simulink model "new_foc_mmd"  (R2024b)
settings: Solver=VariableStepAuto  StartTime=0.0  StopTime=3.14  FixedStep=0.000001  MaxStep=1e-4  RelTol=1e-3
model workspace (MAT data in the model file):
  fs = 4000
undefined symbols (not defined in the file): speed_ref, Ts
libraries: simulink x13, spsIGBTDiodeLib x6, slpidlib x3, spsVoltageMeasurementLib x3, spsPermanentMagnetSynchronousMachineLib x1, spsDCVoltageSourceLib x1, spsSawtoothGeneratorLib x1, simulink_extras x1, spsThreePhaseVIMeasurementLib x1, spspowerguiLib x1
(part 1 of 2)
settings Model: Creator=Admin  LastModifiedBy=INNAGOL2
settings SolverCC: ZeroCrossAlgorithm=Adaptive
settings DebuggingCC: MaskedZcDiagnostic=none  IgnoredZcDiagnostic=none
settings RTWCC: GPUComputeCapability=3.5

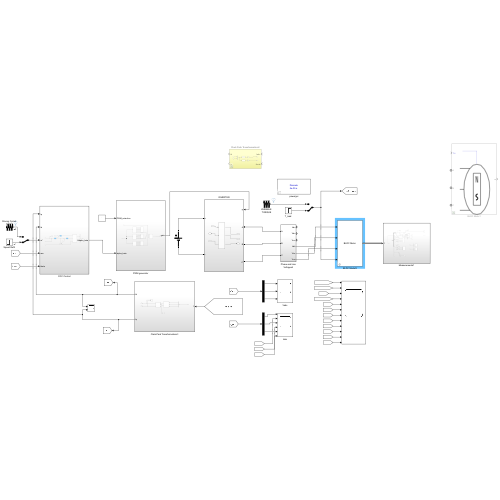
[thumbnail: Simulink's stored preview of the top-level diagram]
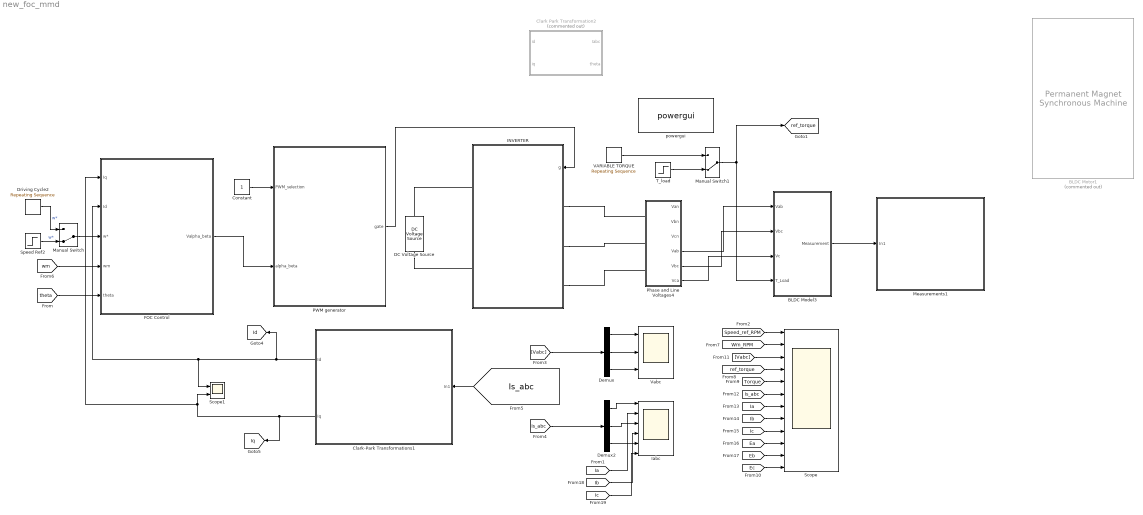
== system new_foc_mmd ==
  BLDC Model3 : Subsystem  mask(BLDC Motor :){Rs=0.7, Lls=2.7e-3, Phi_m=0.1194, J=0.0027, B=0.0004924, P=8}
      mask prompts: Rs "Resistance - Rs [ohms]"; Lls "Inductance - Lls [H]"; Phi_m "Rotor Flux [wb]"; J "Rotor Inertia - J [kg-m^2]"; B "Friction Coefficient -B"; P "No of Poles"
      mask init:
      | Trap=0.5;
      mask Display: fprintf('BLDC Motor')
  BLDC Motor1 : spsPermanentMagnetSynchronousMachineLib/Permanent Magnet Synchronous Machine  Commented=on  NbPhases=3  FluxDistribution=Trapezoidal  RotorType=Round  MechanicalLoad=Torque Tm  PresetModel=No  ShowDetailedParameters=on  MeasurementBus=off  Resistance=0.7  Inductance=2.7e-3  dqInductances=[8.5e-3,8.5e-3]  La=0.000835  MachineConstant=Flux linkage established by magnets (V.s)  Flux=0.1194  VoltageCst=100.0283  TorqueCst=0.9552  Flat=120  Mechanical=[0.0027 0.0004924 4]  PolePairs=4  InitialConditions=[0,0, 0,0]  InitialConditions5ph=[0 0 0 0 0 0]  RefAngle=Aligned with phase A axis (original Park)  IterativeDiscreteModel=Trapezoidal non iterative  TsBlock=-1  TsPowergui=0
  Clark Park Transformation2 : Subsystem  Commented=on
  Clark-Park Transformations1 : Subsystem
      settings: PortSchema="{\"entries\":[{\"content\":{\"sides\":[{\"content\":{\"connectorIds\":[\"Out1\",\"Out2\"]},\"type\":\"ConnectorPlacement.EquallySpacedRectSide\",\"uuid\":\"c290a13d-b4ce-440f-9d53-4b9274feb83f\"},{\"content\":{\"connectorIds\":[\"In1\"],\"side\":\"RIGHT\"},\"type\":\"ConnectorPlacement.EquallySpacedRectSide\",\"uuid\":\"3b8acf4d-0134-48df-ade6-fa9dd8548719\"},{\"content\":{\"side\":\"TOP\"},\"type\":\"ConnectorPlacement.EquallySpacedRectSide\",\"uuid\":\"08682ee2-bcb7-4f48-a64a-1997ed6d0a04\"}]},\"type\":\"ConnectorPlacement.EquallySpacedConnector\",\"uuid\":\"e640fd84-78ba-4bab-8695-1c4b1b64123a\"}],\"packageUris\":[\"http://schema.mathworks.com/mf0/Connector/R2020b\"],\"version\":\"1.0\"}"
  Constant : Constant
  DC Voltage Source : spsDCVoltageSourceLib/DC Voltage Source  Amplitude=160  Measurements=None
  Demux : Demux  Outputs=3
  Demux2 : Demux  Outputs=3
  Driving Cycle2 : simulink/Sources/Repeating Sequence  rep_seq_t=[0 1 2 3 4 5 6 7 8 9 10 11 11.0001 12 13]  rep_seq_y=[0 20 20 0 0 0 -30 -30 0 0 50 50 40 40 0]
  FOC Control : Subsystem
  INVERTER : Subsystem
  Iabc : Scope  NumInputPorts=6
  Manual Switch : ManualSwitch  CurrentSetting=0
  Manual Switch1 : ManualSwitch  CurrentSetting=0
  Measurements1 : Subsystem
  PWM generator : Subsystem
  Phase and Line Voltages4 : Subsystem
  Scope : Scope  NumInputPorts=12
  Scope1 : Scope  NumInputPorts=2
  Speed Ref2 : Step  Time=0.1  After=150  SampleTime=0
  "T_load " : Step  Time=0.1  After=5  SampleTime=0
  VARIABLE TORQUE : simulink/Sources/Repeating Sequence  rep_seq_t=[0 1 2 3 4 5 6 7 8 9 10 11 12 13]  rep_seq_y=[3 3 3 3 5 5 5 -2 -2 -2 1 1 1 1 ]
  Vabc : Scope  NumInputPorts=3
  powergui : spspowerguiLib/powergui  Priority=1  SimulationMode=Discrete  SampleTime=5e-05  frequency=60  Iterations=50  frequencyindice=0  Pbase=100e6  ErrMax=1e-4  UnitsV=kV  UnitsW=MW  buscounter=0  FunctionMessages=off  echomessages=off  EnableUseOfTLC=off  CurrentSourceSwitches=off  DisableSnubberDevices=off  DisableRonSwitches=off  DisableVfSwitches=off  DisplayEquations=off  AutomaticDiscreteSolvers=off  SolverType=Tustin/Backward Euler (TBE)  Interpol=off  ExternalGateDelay=off  methode=off  Ts=100  x0status=blocks  SPID=on  SwTol=0  HookPort=off  NonlinearTolerance=1e-4  nMaxIteration=100  ContinueOnMaxIteration=off  RestoreLinks=warning  ResistiveCurrentMeasurement=off  Frange=[0:2:500]  Ylog=off  Xlog=on  ShowGrid=off  save=off  variable=ZData  structure=0  ZoomFFT=off  StartTime=0.0  cycles=1  DisplayStyle=1  fundamental=60  FreqAxis=off  MaxFrequency=1000  frequencyindicesteady=1  RmsSteady=1  display=off
  tag scope: Id=global, Iq=global, ref_torque=global
  wires:
  Demux/3 -> Vabc/3
  Demux/1 -> Vabc/1
  Demux/2 -> Vabc/2
  Demux2/1 -> Iabc/1
  Demux2/2 -> Iabc/3
  Demux2/3 -> Iabc/5
  [Vabc] -> Demux/1
  [Is_abc] -> Demux2/1
  PWM generator/1(gate) -> INVERTER/1(g)
  [Is_abc] -> Clark-Park Transformations1/1(In1)
  Clark-Park Transformations1/1(Id) -> [Id], Scope1/1, FOC Control/2(Id)
  Clark-Park Transformations1/2(Iq) -> Scope1/2, FOC Control/1(Iq), [Iq]
  [wm] -> FOC Control/4(wm)
  [theta] -> FOC Control/5(theta)
  Constant/1 -> PWM generator/1(PWM_selection)
  FOC Control/1(Valpha_beta) -> PWM generator/2(alpha_beta)
  Speed Ref2/1 -> Manual Switch/2  "w*"
  Manual Switch/1 -> FOC Control/3(w*)
  VARIABLE TORQUE/1 -> Manual Switch1/1
  "T_load "/1 -> Manual Switch1/2
  Manual Switch1/1 -> BLDC Model3/4(T_Load), [ref_torque]
  Driving Cycle2/1 -> Manual Switch/1  "w*"
  [Vabc] -> Scope/3
  [Ib] -> Scope/8
  [Ia] -> Scope/7
  [Ea] -> Scope/10
  [ref_torque] -> Scope/4
  [Ic] -> Scope/9
  [Ec] -> Scope/12
  [Eb] -> Scope/11
  [Torque] -> Scope/5
  [Wm_RPM] -> Scope/2
  [Is_abc] -> Scope/6
  [Speed_ref_RPM] -> Scope/1
  [Ia] -> Iabc/2
  [Ib] -> Iabc/4
  [Ic] -> Iabc/6
  BLDC Model3/1(Measurement) -> Measurements1/1(In1)
  Phase and Line Voltages4/4(Vab) -> BLDC Model3/1(Vab)
  Phase and Line Voltages4/5(Vbc) -> BLDC Model3/2(Vbc)
  Phase and Line Voltages4/6(Vca) -> BLDC Model3/3(Vc)
  connections:
  INVERTER/LConn1 -- Phase and Line Voltages4/LConn1
  DC Voltage Source/RConn1 -- INVERTER/RConn1
  INVERTER/LConn2 -- Phase and Line Voltages4/LConn2
  DC Voltage Source/LConn1 -- INVERTER/RConn2
  INVERTER/LConn3 -- Phase and Line Voltages4/LConn3

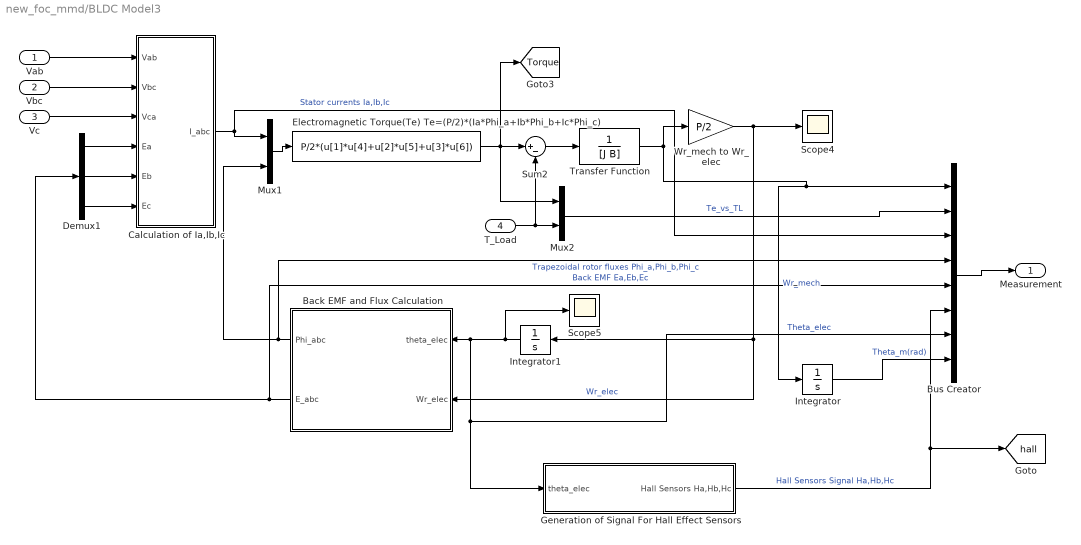
== system new_foc_mmd/BLDC Model3 ==
  Vab : Inport
  Vbc : Inport  Port=2
  Vc : Inport  Port=3
  T_Load : Inport  Port=4
  Back EMF and Flux Calculation : Subsystem
  Bus Creator : BusCreator  Inputs=8
  Calculation of Ia,Ib,Ic : Subsystem
  Demux1 : Demux  Outputs=3
  Electromagnetic Torque(Te) Te=(P/2)*(Ia*Phi_a+Ib*Phi_b+Ic*Phi_c) : Fcn  Expr=P/2*(u[1]*u[4]+u[2]*u[5]+u[3]*u[6])
  Generation of Signal For Hall Effect Sensors : Subsystem
  Integrator : Integrator  WrapState=on
  Integrator1 : Integrator  WrapState=on
  Mux1 : Mux  Inputs=2
  Mux2 : Mux  Inputs=2
  Scope4 : Scope
  Scope5 : Scope
  Sum2 : Sum  Inputs=|+-
  Transfer Function : TransferFcn  Denominator=[J B]
  Wr_mech to Wr_elec : Gain  Gain=P/2
  Measurement : Outport
  tag scope: Torque=global, hall=global
  wires:
  Vc/1 -> Calculation of Ia,Ib,Ic/3(Vca)
  Vab/1 -> Calculation of Ia,Ib,Ic/1(Vab)
  Vbc/1 -> Calculation of Ia,Ib,Ic/2(Vbc)
  Sum2/1 -> Transfer Function/1
  Mux1/1 -> Electromagnetic Torque(Te) Te=(P/2)*(Ia*Phi_a+Ib*Phi_b+Ic*Phi_c)/1
  Demux1/3 -> Calculation of Ia,Ib,Ic/6(Ec)
  Demux1/2 -> Calculation of Ia,Ib,Ic/5(Eb)
  Demux1/1 -> Calculation of Ia,Ib,Ic/4(Ea)
  Integrator1/1 -> Bus Creator/7, Generation of Signal For Hall Effect Sensors/1(theta_elec), Back EMF and Flux Calculation/1(theta_elec), Scope5/1  "Theta_elec"
  Bus Creator/1 -> Measurement/1
  Transfer Function/1 -> Wr_mech to Wr_elec/1, Integrator/1, Bus Creator/1  "Wr_mech"
  Back EMF and Flux Calculation/2(E_abc) -> Bus Creator/5, Demux1/1  "Back EMF Ea,Eb,Ec"
  Wr_mech to Wr_elec/1 -> Back EMF and Flux Calculation/2(Wr_elec), Integrator1/1, Scope4/1  "Wr_elec"
  Back EMF and Flux Calculation/1(Phi_abc) -> Mux1/2, Bus Creator/4  "Trapezoidal rotor fluxes Phi_a,Phi_b,Phi_c"
  Calculation of Ia,Ib,Ic/1(I_abc) -> Mux1/1, Bus Creator/3  "Stator currents Ia,Ib,Ic"
  Electromagnetic Torque(Te) Te=(P/2)*(Ia*Phi_a+Ib*Phi_b+Ic*Phi_c)/1 -> [Torque], Mux2/1, Sum2/1
  Generation of Signal For Hall Effect Sensors/1(Hall Sensors Ha,Hb,Hc) -> [hall], Bus Creator/6  "Hall Sensors Signal Ha,Hb,Hc"
  Mux2/1 -> Bus Creator/2  "Te_vs_TL"
  T_Load/1 -> Sum2/2, Mux2/2
  Integrator/1 -> Bus Creator/8  "Theta_m(rad)"

== system new_foc_mmd/Clark Park Transformation2 ==
  Iabc : Inport
  theta : Inport  Port=2
  Gain : Gain  Gain=2/3
  Gain2 : Gain  Gain=-2/3
  Mux : Mux  Inputs=2
  "iabc -> id" : Fcn  Expr=u(1) * sin(u(4)) + u(2) *sin(u(4) - 2*pi/3) + u(3)*sin(u(4)+2*pi/3)
  "iabc -> iq" : Fcn  Expr=u(1) * cos(u(4)) + u(2) *cos(u(4) - 2*pi/3) + u(3)*cos(u(4)+2*pi/3)
  id : Outport
  iq : Outport  Port=2
  wires:
  Mux/1 -> "iabc -> iq"/1, "iabc -> id"/1
  "iabc -> id"/1 -> Gain2/1
  "iabc -> iq"/1 -> Gain/1
  Iabc/1 -> Mux/1
  theta/1 -> Mux/2
  Gain/1 -> id/1
  Gain2/1 -> iq/1

== system new_foc_mmd/Clark-Park Transformations1 ==
  In1 : Inport
  Clark Transformation : Subsystem
  Demux1 : Demux  Outputs=3
  Park Transformation : Subsystem
  Scope3 : Scope  NumInputPorts=2
  Id : Outport
  Iq : Outport  Port=2
  wires:
  In1/1 -> Demux1/1
  Clark Transformation/1(I_alpha) -> Park Transformation/1(I_alpha)
  Demux1/3 -> Clark Transformation/3(Ic)
  Clark Transformation/2(I_beta) -> Park Transformation/2(I_beta)
  Demux1/2 -> Clark Transformation/2(Ib)
  [theta] -> Park Transformation/3(theta)
  Park Transformation/1(Id) -> Scope3/1, Id/1  "Id"
  Demux1/1 -> Clark Transformation/1(Ia)
  Park Transformation/2(Iq) -> Scope3/2, Iq/1  "Iq"

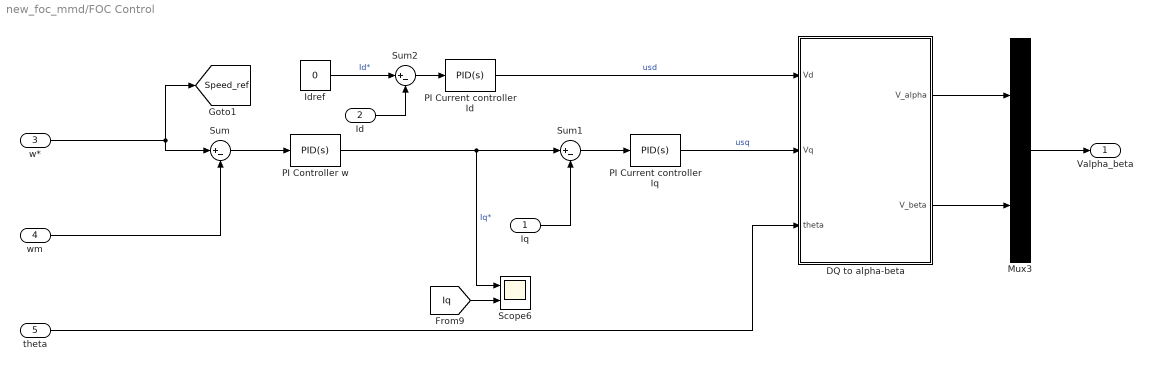
== system new_foc_mmd/FOC Control ==
  Iq : Inport
  Id : Inport  Port=2
  w* : Inport  Port=3
  wm : Inport  Port=4
  theta : Inport  Port=5
  DQ to alpha-beta : Subsystem
  Idref : Constant  Value=0
  Mux3 : Mux  Inputs=2
  PI Controller w : slpidlib/PID Controller  Controller=PID  Form=Parallel  TimeDomain=Continuous-time  UseExternalTs=off  SampleTime=-1  IntegratorMethod=Forward Euler  FilterMethod=Forward Euler  ControllerParametersSource=internal  P=0.00156867  I=0.008414  UseKiTs=off  D=0  UseExternalDerivativeSource=off  N=100  UseFilter=on  TunerSelectOption=Frequency Response Based  InitialConditionSource=internal  InitialConditionForIntegrator=0  InitialConditionForFilter=0  DifferentiatorICPrevScaledInput=0  ExternalReset=none  TrackingMode=off  Kt=1  LimitOutput=on  SatLimitsSource=internal  UpperSaturationLimit=60  LowerSaturationLimit=-60  LinearizeAsGain=on  AntiWindupMode=none  Kb=1  LimitIntegrator=on  UpperIntegratorSaturationLimit=60  LowerIntegratorSaturationLimit=-60  POutMin=[]  POutMax=[]  IOutMin=[]  IOutMax=[]  DOutMin=[]  DOutMax=[]  NOutMin=[]  NOutMax=[]  SumOutMin=[]  SumOutMax=[]  SaturationOutMin=[]  SaturationOutMax=[]  PParamMin=[]  PParamMax=[]  IParamMin=[]  IParamMax=[]  DParamMin=[]  DParamMax=[]  NParamMin=[]  NParamMax=[]  KbParamMin=[]  KbParamMax=[]  KtParamMin=[]  KtParamMax=[]  KbOutMin=[]  KbOutMax=[]  KtOutMin=[]  KtOutMax=[]  IntegratorOutMin=[]  IntegratorOutMax=[]  FilterOutMin=[]  FilterOutMax=[]  SumI1OutMin=[]  SumI1OutMax=[]  SumI2OutMin=[]  SumI2OutMax=[]  SumI3OutMin=[]  SumI3OutMax=[]  SumI4OutMin=[]  SumI4OutMax=[]  SumDOutMin=[]  SumDOutMax=[]  DifferentiatorOutMin=[]  DifferentiatorOutMax=[]  FilterDiffOutCoefMin=[]  FilterDiffOutCoefMax=[]  ReciprocalOutMin=[]  ReciprocalOutMax=[]  SumDenOutMin=[]  SumDenOutMax=[]  SumNumOutMin=[]  SumNumOutMax=[]  DivideOutMin=[]  DivideOutMax=[]  UdiffTsProdOutMin=[]  UdiffTsProdOutMax=[]  NTsProdOutMin=[]  NTsProdOutMax=[]  UintegralTsProdOutMin=[]  UintegralTsProdOutMax=[]  UngainTsProdOutMin=[]  UngainTsProdOutMax=[]  ClampingZeroOutDataTypeStr=Inherit: Inherit via back propagation  ClampingZeroOutMin=[]  ClampingZeroOutMax=[]  FilterDenConstantOutDataTypeStr=Inherit: Inherit via back propagation  FilterDenConstantOutMin=[]  FilterDenConstantOutMax=[]  PCopyOutDataTypeStr=Inherit: Inherit via back propagation  PCopyOutMin=[]  PCopyOutMax=[]  NCopyOutDataTypeStr=Inherit: Inherit via back propagation  NCopyOutMin=[]  NCopyOutMax=[]  IntegratorContinuousStateAttributes=''  IntegratorStateMustResolveToSignalObject=off  IntegratorRTWStateStorageClass=Auto  FilterContinuousStateAttributes=''  FilterStateMustResolveToSignalObject=off  FilterRTWStateStorageClass=Auto  ParallelPVariant=InternalParameters  IdealPVariant=Disabled  IVariant=InternalParameters  DVariant=InternalParameters  IntegratorVariant=Continuous  SatVariant=Enabled  AWVariant=Passthrough  PCopyVariant=Disabled  TRVariant=Disabled  FdbkBlocksVariant=Forward  IdealPFdbkVariant=Disabled  SatFdbkVariant=Disabled  DerivativeFilterVariant=ContFilter  NVariant=InternalParameters  NCopyVariant=Disabled  FilterICVariant=InternalICsFilter  IntegratorICVariant=InternalICs  ExternalResetVariant=Disabled  TRSumVariant=Passthrough  SumFdbkVariant=Disabled  SumVariant=Sum_PID  TsampFilterVariant=InternalTs  TsampNgainVariant=Passthrough  TsampIntegralVariant=Disabled_SignalSpec  ExternalSaturationOutDataTypeStr=Inherit: Same as second input  DerivativeSourceVariant=ErrorSignal  PreIntVariant=InternalPreInt
  PI Current controller Id : slpidlib/PID Controller  Controller=PID  Form=Parallel  TimeDomain=Continuous-time  UseExternalTs=off  SampleTime=-1  IntegratorMethod=Forward Euler  FilterMethod=Forward Euler  ControllerParametersSource=internal  P=350  I=100000  UseKiTs=off  D=0  UseExternalDerivativeSource=off  N=100  UseFilter=on  TunerSelectOption=Transfer Function Based (PID Tuner App)  InitialConditionSource=internal  InitialConditionForIntegrator=0  InitialConditionForFilter=0  DifferentiatorICPrevScaledInput=0  ExternalReset=none  TrackingMode=off  Kt=1  LimitOutput=on  SatLimitsSource=internal  UpperSaturationLimit=600  LowerSaturationLimit=-600  LinearizeAsGain=on  AntiWindupMode=clamping  Kb=1  LimitIntegrator=off  UpperIntegratorSaturationLimit=inf  LowerIntegratorSaturationLimit=-inf  POutMin=[]  POutMax=[]  IOutMin=[]  IOutMax=[]  DOutMin=[]  DOutMax=[]  NOutMin=[]  NOutMax=[]  SumOutMin=[]  SumOutMax=[]  SaturationOutMin=[]  SaturationOutMax=[]  PParamMin=[]  PParamMax=[]  IParamMin=[]  IParamMax=[]  DParamMin=[]  DParamMax=[]  NParamMin=[]  NParamMax=[]  KbParamMin=[]  KbParamMax=[]  KtParamMin=[]  KtParamMax=[]  KbOutMin=[]  KbOutMax=[]  KtOutMin=[]  KtOutMax=[]  IntegratorOutMin=[]  IntegratorOutMax=[]  FilterOutMin=[]  FilterOutMax=[]  SumI1OutMin=[]  SumI1OutMax=[]  SumI2OutMin=[]  SumI2OutMax=[]  SumI3OutMin=[]  SumI3OutMax=[]  SumI4OutMin=[]  SumI4OutMax=[]  SumDOutMin=[]  SumDOutMax=[]  DifferentiatorOutMin=[]  DifferentiatorOutMax=[]  FilterDiffOutCoefMin=[]  FilterDiffOutCoefMax=[]  ReciprocalOutMin=[]  ReciprocalOutMax=[]  SumDenOutMin=[]  SumDenOutMax=[]  SumNumOutMin=[]  SumNumOutMax=[]  DivideOutMin=[]  DivideOutMax=[]  UdiffTsProdOutMin=[]  UdiffTsProdOutMax=[]  NTsProdOutMin=[]  NTsProdOutMax=[]  UintegralTsProdOutMin=[]  UintegralTsProdOutMax=[]  UngainTsProdOutMin=[]  UngainTsProdOutMax=[]  ClampingZeroOutDataTypeStr=Inherit: Inherit via back propagation  ClampingZeroOutMin=[]  ClampingZeroOutMax=[]  FilterDenConstantOutDataTypeStr=Inherit: Inherit via back propagation  FilterDenConstantOutMin=[]  FilterDenConstantOutMax=[]  PCopyOutDataTypeStr=Inherit: Inherit via back propagation  PCopyOutMin=[]  PCopyOutMax=[]  NCopyOutDataTypeStr=Inherit: Inherit via back propagation  NCopyOutMin=[]  NCopyOutMax=[]  IntegratorContinuousStateAttributes=''  IntegratorStateMustResolveToSignalObject=off  IntegratorRTWStateStorageClass=Auto  FilterContinuousStateAttributes=''  FilterStateMustResolveToSignalObject=off  FilterRTWStateStorageClass=Auto  ParallelPVariant=InternalParameters  IdealPVariant=Disabled  IVariant=InternalParameters  DVariant=InternalParameters  IntegratorVariant=Continuous  SatVariant=Enabled  AWVariant=ContClampingParallel  PCopyVariant=Disabled  TRVariant=Disabled  FdbkBlocksVariant=Forward  IdealPFdbkVariant=Disabled  SatFdbkVariant=Disabled  DerivativeFilterVariant=ContFilter  NVariant=InternalParameters  NCopyVariant=Disabled  FilterICVariant=InternalICsFilter  IntegratorICVariant=InternalICs  ExternalResetVariant=Disabled  TRSumVariant=Passthrough  SumFdbkVariant=Disabled  SumVariant=Sum_PID  TsampFilterVariant=InternalTs  TsampNgainVariant=Passthrough  TsampIntegralVariant=Disabled_SignalSpec  ExternalSaturationOutDataTypeStr=Inherit: Same as second input  DerivativeSourceVariant=ErrorSignal  PreIntVariant=InternalPreInt
  PI Current controller Iq : slpidlib/PID Controller  Controller=PID  Form=Parallel  TimeDomain=Continuous-time  UseExternalTs=off  SampleTime=-1  IntegratorMethod=Forward Euler  FilterMethod=Forward Euler  ControllerParametersSource=internal  P=350  I=100000  UseKiTs=off  D=0  UseExternalDerivativeSource=off  N=100  UseFilter=on  TunerSelectOption=Transfer Function Based (PID Tuner App)  InitialConditionSource=internal  InitialConditionForIntegrator=0  InitialConditionForFilter=0  DifferentiatorICPrevScaledInput=0  ExternalReset=none  TrackingMode=off  Kt=1  LimitOutput=on  SatLimitsSource=internal  UpperSaturationLimit=600  LowerSaturationLimit=-600  LinearizeAsGain=on  AntiWindupMode=clamping  Kb=1  LimitIntegrator=off  UpperIntegratorSaturationLimit=inf  LowerIntegratorSaturationLimit=-inf  POutMin=[]  POutMax=[]  IOutMin=[]  IOutMax=[]  DOutMin=[]  DOutMax=[]  NOutMin=[]  NOutMax=[]  SumOutMin=[]  SumOutMax=[]  SaturationOutMin=[]  SaturationOutMax=[]  PParamMin=[]  PParamMax=[]  IParamMin=[]  IParamMax=[]  DParamMin=[]  DParamMax=[]  NParamMin=[]  NParamMax=[]  KbParamMin=[]  KbParamMax=[]  KtParamMin=[]  KtParamMax=[]  KbOutMin=[]  KbOutMax=[]  KtOutMin=[]  KtOutMax=[]  IntegratorOutMin=[]  IntegratorOutMax=[]  FilterOutMin=[]  FilterOutMax=[]  SumI1OutMin=[]  SumI1OutMax=[]  SumI2OutMin=[]  SumI2OutMax=[]  SumI3OutMin=[]  SumI3OutMax=[]  SumI4OutMin=[]  SumI4OutMax=[]  SumDOutMin=[]  SumDOutMax=[]  DifferentiatorOutMin=[]  DifferentiatorOutMax=[]  FilterDiffOutCoefMin=[]  FilterDiffOutCoefMax=[]  ReciprocalOutMin=[]  ReciprocalOutMax=[]  SumDenOutMin=[]  SumDenOutMax=[]  SumNumOutMin=[]  SumNumOutMax=[]  DivideOutMin=[]  DivideOutMax=[]  UdiffTsProdOutMin=[]  UdiffTsProdOutMax=[]  NTsProdOutMin=[]  NTsProdOutMax=[]  UintegralTsProdOutMin=[]  UintegralTsProdOutMax=[]  UngainTsProdOutMin=[]  UngainTsProdOutMax=[]  ClampingZeroOutDataTypeStr=Inherit: Inherit via back propagation  ClampingZeroOutMin=[]  ClampingZeroOutMax=[]  FilterDenConstantOutDataTypeStr=Inherit: Inherit via back propagation  FilterDenConstantOutMin=[]  FilterDenConstantOutMax=[]  PCopyOutDataTypeStr=Inherit: Inherit via back propagation  PCopyOutMin=[]  PCopyOutMax=[]  NCopyOutDataTypeStr=Inherit: Inherit via back propagation  NCopyOutMin=[]  NCopyOutMax=[]  IntegratorContinuousStateAttributes=''  IntegratorStateMustResolveToSignalObject=off  IntegratorRTWStateStorageClass=Auto  FilterContinuousStateAttributes=''  FilterStateMustResolveToSignalObject=off  FilterRTWStateStorageClass=Auto  ParallelPVariant=InternalParameters  IdealPVariant=Disabled  IVariant=InternalParameters  DVariant=InternalParameters  IntegratorVariant=Continuous  SatVariant=Enabled  AWVariant=ContClampingParallel  PCopyVariant=Disabled  TRVariant=Disabled  FdbkBlocksVariant=Forward  IdealPFdbkVariant=Disabled  SatFdbkVariant=Disabled  DerivativeFilterVariant=ContFilter  NVariant=InternalParameters  NCopyVariant=Disabled  FilterICVariant=InternalICsFilter  IntegratorICVariant=InternalICs  ExternalResetVariant=Disabled  TRSumVariant=Passthrough  SumFdbkVariant=Disabled  SumVariant=Sum_PID  TsampFilterVariant=InternalTs  TsampNgainVariant=Passthrough  TsampIntegralVariant=Disabled_SignalSpec  ExternalSaturationOutDataTypeStr=Inherit: Same as second input  DerivativeSourceVariant=ErrorSignal  PreIntVariant=InternalPreInt
  Scope6 : Scope  NumInputPorts=2
  Sum : Sum  Inputs=|+-
  Sum1 : Sum  Inputs=|+-
  Sum2 : Sum  Inputs=|+-
  Valpha_beta : Outport
  tag scope: Speed_ref=global
  wires:
  PI Current controller Iq/1 -> DQ to alpha-beta/2(Vq)  "usq"
  PI Controller w/1 -> Scope6/1, Sum1/1  "Iq*"
  theta/1 -> DQ to alpha-beta/3(theta)
  Idref/1 -> Sum2/1  "Id*"
  Sum1/1 -> PI Current controller Iq/1
  Sum2/1 -> PI Current controller Id/1
  Sum/1 -> PI Controller w/1
  w*/1 -> [Speed_ref], Sum/1
  [Iq] -> Scope6/2
  PI Current controller Id/1 -> DQ to alpha-beta/1(Vd)  "usd"
  DQ to alpha-beta/1(V_alpha) -> Mux3/1
  DQ to alpha-beta/2(V_beta) -> Mux3/2
  Mux3/1 -> Valpha_beta/1
  Iq/1 -> Sum1/2
  wm/1 -> Sum/2
  Id/1 -> Sum2/2

== system new_foc_mmd/INVERTER ==
  g : Inport
  Subsystem1 : Subsystem
  A : PMIOPort  Side=Left
  B : PMIOPort  Port=2  Side=Left
  C : PMIOPort  Port=3  Side=Left
  + : PMIOPort  Port=4  Side=Right
  - : PMIOPort  Port=5  Side=Right
  wires:
  g/1 -> Subsystem1/1(Gate)
  connections:
  +/RConn1 -- Subsystem1/LConn1
  -/RConn1 -- Subsystem1/LConn2
  C/RConn1 -- Subsystem1/RConn3
  B/RConn1 -- Subsystem1/RConn2
  A/RConn1 -- Subsystem1/RConn1

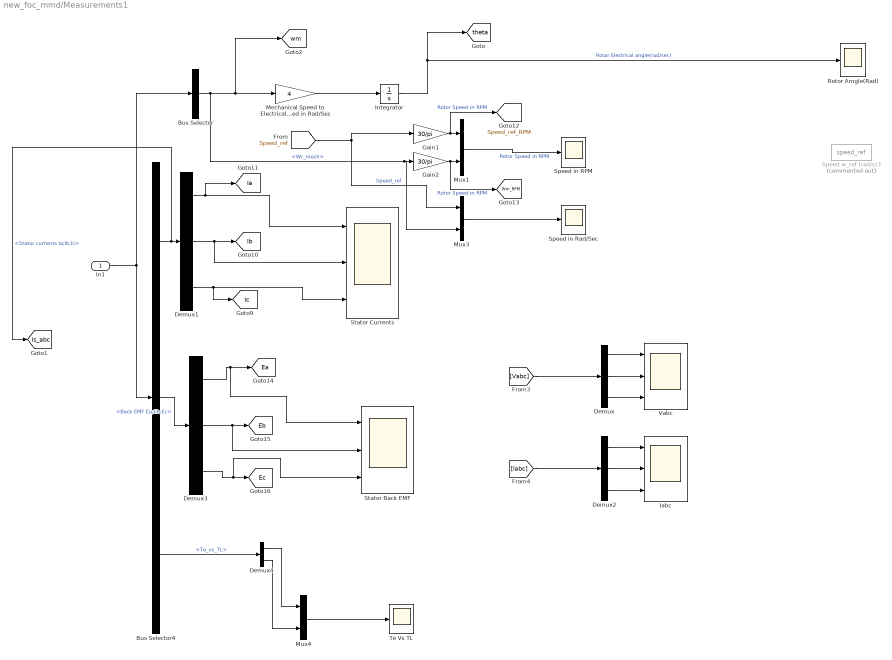
== system new_foc_mmd/Measurements1 ==
  In1 : Inport
  Bus Selector : BusSelector  OutputSignals=Wr_mech
  Bus Selector4 : BusSelector  OutputSignals=|
      | Stator currents
      | Ia;Ib;Ic,Back EMF
      | Ea;Eb;Ec,Te_vs_TL
  Demux{,1..3} (4 alike) : Demux  Outputs=3
  Demux4 : Demux  Outputs=2
  Gain1 : Gain  Gain=30/pi
  Gain2 : Gain  Gain=30/pi
  Iabc : Scope  NumInputPorts=3
  Integrator : Integrator  WrapState=on
  Mechanical Speed to Electrical speed in Rad/Sec : Gain  Gain=4
  Mux1 : Mux  Inputs=2
  Mux3 : Mux  Inputs=2
  Mux4 : Mux  Inputs=2
  Rotor Amgle(Rad) : Scope
  Speed in RPM : Scope
  Speed in Rad/Sec : Scope
  Speed w_ref (rad/s)3 : Constant  Commented=on  Value=speed_ref
  Stator Back EMF : Scope  NumInputPorts=3
  Stator Currents : Scope  NumInputPorts=3
  Te Vs TL : Scope
  Vabc : Scope  NumInputPorts=3
  tag scope: Ea=global, Eb=global, Ec=global, Ia=global, Ib=global, Ic=global, Is_abc=global, Speed_ref_RPM=global, Wm_RPM=global, theta=global, wm=global
  wires:
  Demux/1 -> Vabc/1
  [Iabc] -> Demux2/1
  Demux2/2 -> Iabc/2
  Demux/3 -> Vabc/3
  Demux2/1 -> Iabc/1
  [Vabc] -> Demux/1
  Demux2/3 -> Iabc/3
  Demux/2 -> Vabc/2
  Gain2/1 -> Mux1/2, [Wm_RPM]  "Rotor Speed in RPM"
  In1/1 -> Bus Selector/1, Bus Selector4/1
  Mux1/1 -> Speed in RPM/1  "Rotor Speed in RPM"
  [Speed_ref] -> Gain1/1, Mux3/1  "Speed_ref"
  Mux3/1 -> Speed in Rad/Sec/1
  Mechanical Speed to Electrical speed in Rad/Sec/1 -> Integrator/1
  Gain1/1 -> Mux1/1, [Speed_ref_RPM]  "Rotor Speed in RPM"
  Bus Selector/1 -> Mux3/2, Gain2/1, [wm], Mechanical Speed to Electrical speed in Rad/Sec/1  "<Wr_mech>"
  Integrator/1 -> Rotor Amgle(Rad)/1, [theta]  "Rotar Electrical angle(rad/sec)"
  Mux4/1 -> Te Vs TL/1
  Bus Selector4/1 -> [Is_abc], Demux1/1  "<Stator currents Ia;Ib;Ic>"
  Demux1/1 -> [Ia], Stator Currents/1
  Demux1/2 -> [Ib], Stator Currents/2
  Demux1/3 -> [Ic], Stator Currents/3
  Bus Selector4/2 -> Demux3/1  "<Back EMF Ea;Eb;Ec>"
  Demux3/1 -> Stator Back EMF/1, [Ea]
  Demux3/2 -> Stator Back EMF/2, [Eb]
  Demux3/3 -> Stator Back EMF/3, [Ec]
  Bus Selector4/3 -> Demux4/1  "<Te_vs_TL>"
  Demux4/1 -> Mux4/1
  Demux4/2 -> Mux4/2

== system new_foc_mmd/PWM generator ==
  PWM_selection : Inport
  alpha_beta : Inport  Port=2
  Gate : Scope  NumInputPorts=6
  Multiport Switch : MultiPortSwitch  SaturateOnIntegerOverflow=off  InputSameDT=off
  PWM : Subsystem
  SPWM : Subsystem
  SVPWM : Subsystem
  Scope4 : Scope  NumInputPorts=6
  Scope9 : Scope  NumInputPorts=6
  gate : Outport
  wires:
  SVPWM/2(g4) -> Scope9/2
  PWM/2(g4) -> Scope4/2
  PWM/3(g3) -> Scope4/3
  PWM/1(g1) -> Scope4/1
  SPWM/3(g3) -> Gate/3
  SVPWM/1(g1) -> Scope9/1
  alpha_beta/1 -> SPWM/1(alpha_beta), SVPWM/1(alpha beta), PWM/1(alpha_beta)
  SVPWM/3(g3) -> Scope9/3
  PWM/5(g5) -> Scope4/5
  PWM/7(Gate) -> Multiport Switch/4
  PWM/6(g2) -> Scope4/6
  SPWM/5(g5) -> Gate/5
  SPWM/4(g6) -> Gate/4
  SPWM/1(g1) -> Gate/1
  SPWM/2(g4) -> Gate/2
  SPWM/6(g2) -> Gate/6
  SPWM/7(gate) -> Multiport Switch/2
  PWM/4(g6) -> Scope4/4
  PWM_selection/1 -> Multiport Switch/1
  Multiport Switch/1 -> gate/1
  SVPWM/4(g6) -> Scope9/4
  SVPWM/5(g5) -> Scope9/5
  SVPWM/6(g2) -> Scope9/6
  SVPWM/7(Gate1) -> Multiport Switch/3

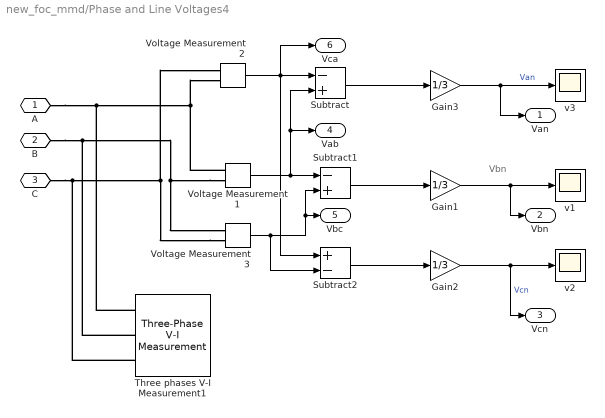
== system new_foc_mmd/Phase and Line Voltages4 ==
  note: Vbn
  Gain1 : Gain  Gain=1/3
  Gain2 : Gain  Gain=1/3
  Gain3 : Gain  Gain=1/3
  Subtract : Sum  Inputs=-+
  Subtract1 : Sum  Inputs=-+
  Subtract2 : Sum  Inputs=+-
  Three phases V-I Measurement1 : spsThreePhaseVIMeasurementLib/Three-Phase V-I Measurement  VoltageMeasurement=phase-to-phase  SetLabelV=on  LabelV=Vabc  Vpu=off  VpuLL=off  CurrentMeasurement=no  SetLabelI=on  LabelI=Iabc  Ipu=off  Pbase=100e6  Vbase=500e3  OutputType=Complex  PhasorSimulation=off  PSBequivalent=0
  Voltage Measurement1 : spsVoltageMeasurementLib/Voltage Measurement  PhasorSimulation=off  OutputType=Complex  PSBequivalent=0
  Voltage Measurement2 : spsVoltageMeasurementLib/Voltage Measurement  PhasorSimulation=off  OutputType=Complex  PSBequivalent=0
  Voltage Measurement3 : spsVoltageMeasurementLib/Voltage Measurement  PhasorSimulation=off  OutputType=Complex  PSBequivalent=0
  v1 : Scope
  v2 : Scope
  v3 : Scope
  A : PMIOPort  Side=Left
  B : PMIOPort  Port=2  Side=Left
  C : PMIOPort  Port=3  Side=Left
  Van : Outport  VectorParamsAs1DForOutWhenUnconnected=off
  Vbn : Outport  Port=2  VectorParamsAs1DForOutWhenUnconnected=off
  Vcn : Outport  Port=3  VectorParamsAs1DForOutWhenUnconnected=off
  Vab : Outport  Port=4  VectorParamsAs1DForOutWhenUnconnected=off
  Vbc : Outport  Port=5  VectorParamsAs1DForOutWhenUnconnected=off
  Vca : Outport  Port=6  VectorParamsAs1DForOutWhenUnconnected=off
  wires:
  Gain2/1 -> v2/1, Vcn/1  "Vcn"
  Subtract2/1 -> Gain2/1
  Gain1/1 -> v1/1, Vbn/1
  Subtract1/1 -> Gain1/1
  Voltage Measurement3/1 -> Subtract1/2, Vbc/1, Subtract2/2
  Gain3/1 -> v3/1, Van/1  "Van"
  Subtract/1 -> Gain3/1
  Voltage Measurement1/1 -> Vab/1, Subtract/2, Subtract1/1
  Voltage Measurement2/1 -> Vca/1, Subtract2/1, Subtract/1
  connections:
  Voltage Measurement1/LConn1 -- Three phases V-I Measurement1/LConn1 -- A/RConn1 -- Voltage Measurement2/LConn2
  Voltage Measurement1/LConn2 -- Three phases V-I Measurement1/LConn2 -- B/RConn1 -- Voltage Measurement3/LConn1
  Voltage Measurement3/LConn2 -- Three phases V-I Measurement1/LConn3 -- C/RConn1 -- Voltage Measurement2/LConn1

== system new_foc_mmd/BLDC Model3/Back EMF and Flux Calculation ==
  theta_elec : Inport
  Wr_elec : Inport  Port=2
  " " : Gain  Gain=Phi_m/Trap
  " " : Gain  Gain=Phi_m/Trap
  " " : Gain  Gain=Phi_m/Trap
  E=Phi_abc*Wr_elec : Product
  Fcn1 : Fcn  Expr=cos(u-2*pi/3)
  Fcn2 : Fcn  Expr=cos(u-4*pi/3)
  Fcn3 : Fcn  Expr=cos(u)
  Mux : Mux  Inputs=3
  Saturation : Saturate  UpperLimit=Trap  LowerLimit=-Trap
  Saturation1 : Saturate  UpperLimit=Trap  LowerLimit=-Trap
  Saturation2 : Saturate  UpperLimit=Trap  LowerLimit=-Trap
  Phi_abc : Outport
  E_abc : Outport  Port=2
  wires:
  Fcn3/1 -> Saturation/1
  theta_elec/1 -> Fcn2/1, Fcn1/1, Fcn3/1
  Fcn2/1 -> Saturation2/1
  Fcn1/1 -> Saturation1/1
  " "/1 -> Mux/1
  " "/1 -> Mux/2
  " "/1 -> Mux/3
  Mux/1 -> Phi_abc/1, E=Phi_abc*Wr_elec/1
  Wr_elec/1 -> E=Phi_abc*Wr_elec/2
  E=Phi_abc*Wr_elec/1 -> E_abc/1
  Saturation/1 -> " "/1
  Saturation1/1 -> " "/1
  Saturation2/1 -> " "/1

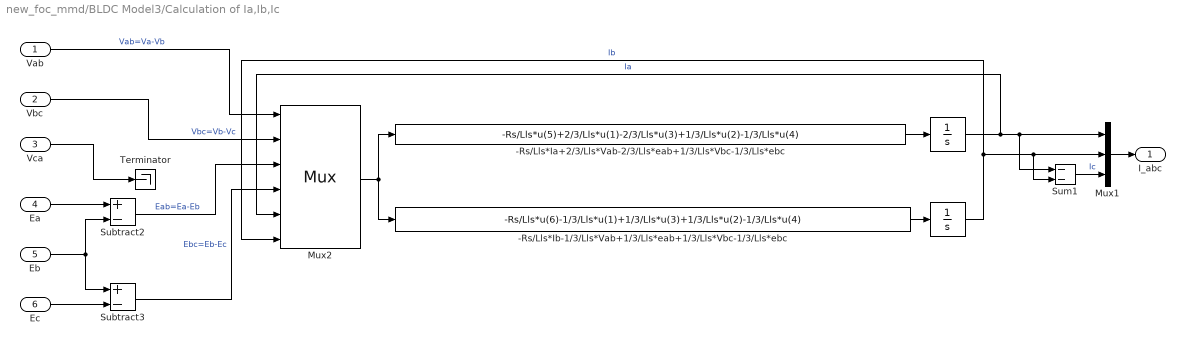
== system new_foc_mmd/BLDC Model3/Calculation of Ia,Ib,Ic ==
  Vab : Inport
  Vbc : Inport  Port=2
  Vca : Inport  Port=3
  Ea : Inport  Port=4
  Eb : Inport  Port=5
  Ec : Inport  Port=6
  " " : Integrator
  " " : Integrator
  -Rs/Lls*Ia+2/3/Lls*Vab-2/3/Lls*eab+1/3/Lls*Vbc-1/3/Lls*ebc : Fcn  Expr=-Rs/Lls*u(5)+2/3/Lls*u(1)-2/3/Lls*u(3)+1/3/Lls*u(2)-1/3/Lls*u(4)
  -Rs/Lls*Ib-1/3/Lls*Vab+1/3/Lls*eab+1/3/Lls*Vbc-1/3/Lls*ebc : Fcn  Expr=-Rs/Lls*u(6)-1/3/Lls*u(1)+1/3/Lls*u(3)+1/3/Lls*u(2)-1/3/Lls*u(4)
  Mux1 : Mux  Inputs=3
  Mux2 : Mux  Inputs=6
      settings: DisplayOption=signals
  Subtract2 : Sum  Inputs=+-
  Subtract3 : Sum  Inputs=+-
  Sum1 : Sum  Inputs=--  SaturateOnIntegerOverflow=on
  Terminator : Terminator
  I_abc : Outport
  wires:
  Eb/1 -> Subtract3/1, Subtract2/2
  Ea/1 -> Subtract2/1
  Ec/1 -> Subtract3/2
  -Rs/Lls*Ia+2/3/Lls*Vab-2/3/Lls*eab+1/3/Lls*Vbc-1/3/Lls*ebc/1 -> " "/1
  Subtract3/1 -> Mux2/4  "Ebc=Eb-Ec"
  -Rs/Lls*Ib-1/3/Lls*Vab+1/3/Lls*eab+1/3/Lls*Vbc-1/3/Lls*ebc/1 -> " "/1
  Vab/1 -> Mux2/1  "Vab=Va-Vb"
  Vbc/1 -> Mux2/2  "Vbc=Vb-Vc"
  Subtract2/1 -> Mux2/3  "Eab=Ea-Eb"
  Mux2/1 -> -Rs/Lls*Ia+2/3/Lls*Vab-2/3/Lls*eab+1/3/Lls*Vbc-1/3/Lls*ebc/1, -Rs/Lls*Ib-1/3/Lls*Vab+1/3/Lls*eab+1/3/Lls*Vbc-1/3/Lls*ebc/1
  " "/1 -> Mux1/2, Sum1/2, Mux2/6  "Ib"
  " "/1 -> Sum1/1, Mux1/1, Mux2/5  "Ia"
  Sum1/1 -> Mux1/3  "Ic"
  Mux1/1 -> I_abc/1
  Vca/1 -> Terminator/1

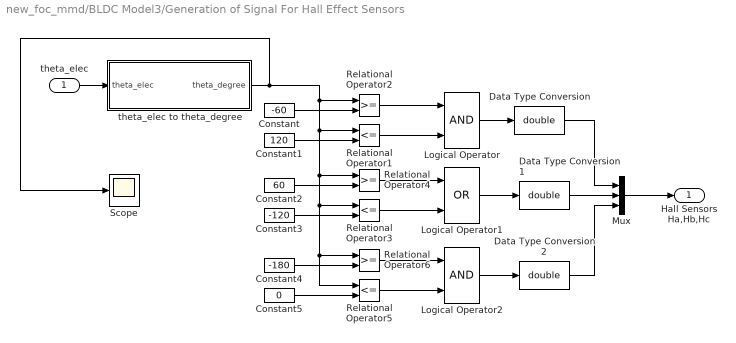
== system new_foc_mmd/BLDC Model3/Generation of Signal For Hall Effect Sensors ==
  theta_elec : Inport
  Constant : Constant  Value=-60
  Constant1 : Constant  Value=120
  Constant2 : Constant  Value=60
  Constant3 : Constant  Value=-120
  Constant4 : Constant  Value=-180
  Constant5 : Constant  Value=0
  Data Type Conversion : DataTypeConversion  OutDataTypeStr=double
  Data Type Conversion1 : DataTypeConversion  OutDataTypeStr=double
  Data Type Conversion2 : DataTypeConversion  OutDataTypeStr=double
  Logical Operator : Logic  AllPortsSameDT=off  OutDataTypeStr=boolean
  Logical Operator1 : Logic  Operator=OR  AllPortsSameDT=off  OutDataTypeStr=boolean
  Logical Operator2 : Logic  AllPortsSameDT=off  OutDataTypeStr=boolean
  Mux : Mux  Inputs=3
  Relational Operator1 : RelationalOperator  Operator=<=
  Relational Operator2 : RelationalOperator
  Relational Operator3 : RelationalOperator  Operator=<=
  Relational Operator4 : RelationalOperator
  Relational Operator5 : RelationalOperator  Operator=<=
  Relational Operator6 : RelationalOperator
  Scope : Scope
  theta_elec to theta_degree : Subsystem
  Hall Sensors Ha,Hb,Hc : Outport
  wires:
  Constant3/1 -> Relational Operator3/2
  Data Type Conversion2/1 -> Mux/3
  Data Type Conversion1/1 -> Mux/2
  Data Type Conversion/1 -> Mux/1
  Relational Operator5/1 -> Logical Operator2/2
  Logical Operator2/1 -> Data Type Conversion2/1
  Relational Operator6/1 -> Logical Operator2/1
  Constant4/1 -> Relational Operator6/2
  Constant5/1 -> Relational Operator5/2
  Relational Operator3/1 -> Logical Operator1/2
  Logical Operator1/1 -> Data Type Conversion1/1
  Logical Operator/1 -> Data Type Conversion/1
  Mux/1 -> Hall Sensors Ha,Hb,Hc/1
  Relational Operator2/1 -> Logical Operator/1
  Relational Operator1/1 -> Logical Operator/2
  Constant/1 -> Relational Operator2/2
  Relational Operator4/1 -> Logical Operator1/1
  Constant1/1 -> Relational Operator1/2
  Constant2/1 -> Relational Operator4/2
  theta_elec/1 -> theta_elec to theta_degree/1(theta_elec)
  theta_elec to theta_degree/1(theta_degree) -> Scope/1, Relational Operator4/1, Relational Operator3/1, Relational Operator5/1, Relational Operator6/1, Relational Operator1/1, Relational Operator2/1

== system new_foc_mmd/Clark-Park Transformations1/Clark Transformation ==
  Ia : Inport
  Ib : Inport  Port=2
  Ic : Inport  Port=3
  Gain : Gain
  Gain1 : Gain  Gain=-1/2
  Gain2 : Gain  Gain=-1/2
  Gain3 : Gain  Gain=(sqrt(3))/2
  Gain4 : Gain  Gain=(-sqrt(3))/2
  Sum3 : Sum  Inputs=|+++
  Sum4 : Sum  Inputs=|++
  I_alpha : Outport
  I_beta : Outport  Port=2
  wires:
  Sum4/1 -> I_beta/1
  Ia/1 -> Gain/1
  Gain4/1 -> Sum4/2
  Gain1/1 -> Sum3/2
  Ic/1 -> Gain2/1, Gain4/1
  Gain/1 -> Sum3/1
  Gain3/1 -> Sum4/1
  Sum3/1 -> I_alpha/1
  Ib/1 -> Gain1/1, Gain3/1
  Gain2/1 -> Sum3/3

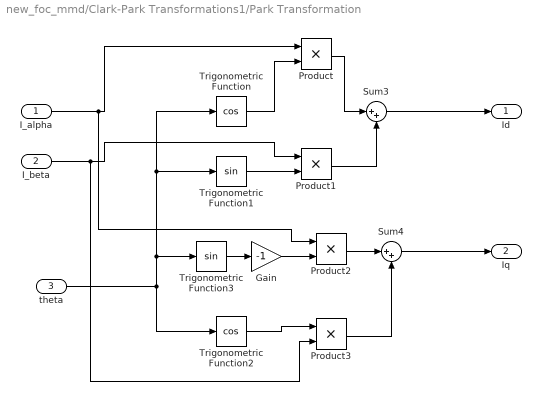
== system new_foc_mmd/Clark-Park Transformations1/Park Transformation ==
  I_alpha : Inport
  I_beta : Inport  Port=2
  theta : Inport  Port=3
  Gain : Gain  Gain=-1
  Product{,1..3} (4 alike) : Product
  Sum3 : Sum  Inputs=|++
  Sum4 : Sum  Inputs=|++
  Trigonometric Function : Trigonometry  Operator=cos
  Trigonometric Function1 : Trigonometry
  Trigonometric Function2 : Trigonometry  Operator=cos
  Trigonometric Function3 : Trigonometry
  Id : Outport
  Iq : Outport  Port=2
  wires:
  Sum4/1 -> Iq/1
  Sum3/1 -> Id/1
  Product3/1 -> Sum4/2
  Product2/1 -> Sum4/1
  Trigonometric Function2/1 -> Product3/1
  Gain/1 -> Product2/2
  Product1/1 -> Sum3/2
  Product/1 -> Sum3/1
  I_beta/1 -> Product1/1, Product3/2
  Trigonometric Function1/1 -> Product1/2
  I_alpha/1 -> Product/1, Product2/1
  Trigonometric Function/1 -> Product/2
  theta/1 -> Trigonometric Function/1, Trigonometric Function1/1, Trigonometric Function3/1, Trigonometric Function2/1
  Trigonometric Function3/1 -> Gain/1

== system new_foc_mmd/FOC Control/DQ to alpha-beta ==
  Vd : Inport
  Vq : Inport  Port=2
  theta : Inport  Port=3
  Product{,1..3} (4 alike) : Product
  Sum3 : Sum  Inputs=|+-
  Sum4 : Sum  Inputs=|++
  Trigonometric Function : Trigonometry  Operator=cos
  Trigonometric Function1 : Trigonometry
  Trigonometric Function2 : Trigonometry  Operator=cos
  Trigonometric Function3 : Trigonometry
  V_alpha : Outport
  V_beta : Outport  Port=2
  wires:
  Product3/1 -> Sum4/2
  Product2/1 -> Sum4/1
  Trigonometric Function2/1 -> Product3/1
  Trigonometric Function3/1 -> Product2/2
  Product1/1 -> Sum3/2
  Product/1 -> Sum3/1
  Vq/1 -> Product1/1, Product3/2
  Trigonometric Function1/1 -> Product1/2
  Vd/1 -> Product/1, Product2/1
  Trigonometric Function/1 -> Product/2
  theta/1 -> Trigonometric Function/1, Trigonometric Function1/1, Trigonometric Function3/1, Trigonometric Function2/1
  Sum4/1 -> V_beta/1
  Sum3/1 -> V_alpha/1

== system new_foc_mmd/INVERTER/Subsystem1 ==
  Gate : Inport
  Demux5 : Demux  Outputs=6
  IGBT/Diode{13..18} (6 alike) : spsIGBTDiodeLib/IGBT//Diode  Ron=1e-3  Rs=1e5  Cs=inf  Measurements=off
  A : PMIOPort  Side=Right
  +ve : PMIOPort  Port=2  Side=Left
  B : PMIOPort  Port=3  Side=Right
  -ve : PMIOPort  Port=4  Side=Left
  C : PMIOPort  Port=5  Side=Right
  wires:
  Demux5/3 -> IGBT/Diode18/1
  Demux5/2 -> IGBT/Diode17/1
  Demux5/6 -> IGBT/Diode15/1
  Demux5/1 -> IGBT/Diode16/1
  Gate/1 -> Demux5/1
  Demux5/4 -> IGBT/Diode14/1
  Demux5/5 -> IGBT/Diode13/1
  connections:
  IGBT/Diode15/LConn1 -- C/RConn1 -- IGBT/Diode13/RConn1
  IGBT/Diode18/RConn1 -- B/RConn1 -- IGBT/Diode14/LConn1
  IGBT/Diode14/RConn1 -- IGBT/Diode17/RConn1 -- -ve/RConn1 -- IGBT/Diode15/RConn1
  IGBT/Diode16/RConn1 -- A/RConn1 -- IGBT/Diode17/LConn1
  IGBT/Diode16/LConn1 -- IGBT/Diode18/LConn1 -- +ve/RConn1 -- IGBT/Diode13/LConn1

== system new_foc_mmd/PWM generator/PWM ==
  alpha_beta : Inport
  Demux2 : Demux  Outputs=6
  Gate Pulse : Subsystem
  Mux : Mux  Inputs=3
  Scope : Scope
  alpha-beta to ABC : Subsystem
  g1 : Outport
  g4 : Outport  Port=2
  g3 : Outport  Port=3
  g6 : Outport  Port=4
  g5 : Outport  Port=5
  g2 : Outport  Port=6
  Gate : Outport  Port=7
  wires:
  Gate Pulse/1(Out1) -> Gate/1, Demux2/1
  alpha-beta to ABC/3(Vc) -> Mux/3
  Demux2/3 -> g3/1
  alpha-beta to ABC/1(Va) -> Scope/1, Mux/1
  Mux/1 -> Gate Pulse/1(gates)
  Demux2/5 -> g5/1
  Demux2/2 -> g4/1
  alpha-beta to ABC/2(Vb) -> Mux/2
  alpha_beta/1 -> alpha-beta to ABC/1(alpha_beta)
  Demux2/6 -> g2/1
  Demux2/4 -> g6/1
  Demux2/1 -> g1/1

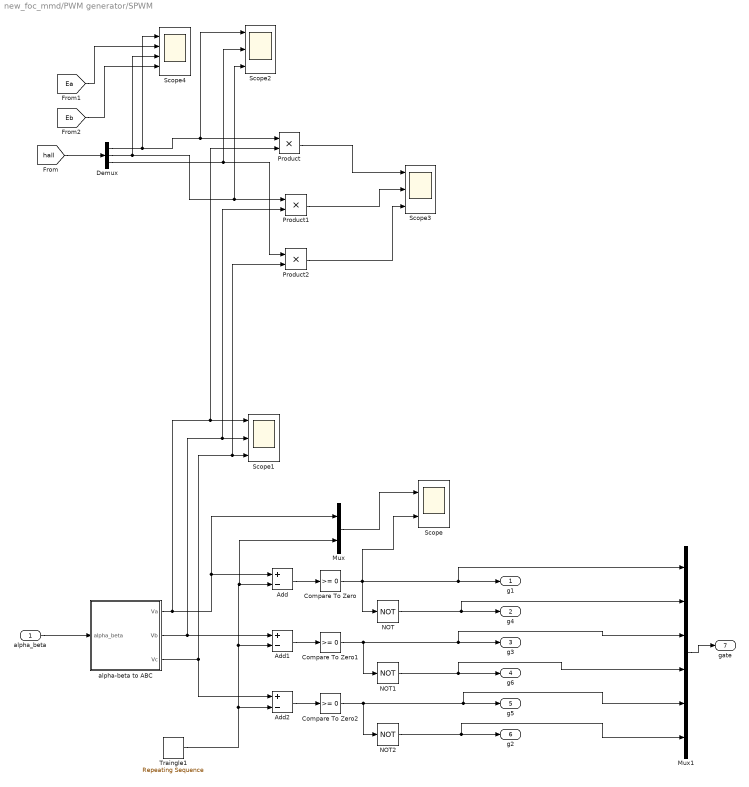
== system new_foc_mmd/PWM generator/SPWM ==
  alpha_beta : Inport
  Add : Sum  Inputs=+-
  Add1 : Sum  Inputs=+-
  Add2 : Sum  Inputs=+-
  Compare To Zero : simulink/Logic and Bit Operations/Compare To Zero  relop=>=  OutDataTypeStr=boolean
  Compare To Zero1 : simulink/Logic and Bit Operations/Compare To Zero  relop=>=  OutDataTypeStr=boolean
  Compare To Zero2 : simulink/Logic and Bit Operations/Compare To Zero  relop=>=  OutDataTypeStr=boolean
  Demux : Demux  Outputs=3
  Mux : Mux  Inputs=2
  Mux1 : Mux  Inputs=6
  NOT : Logic  Operator=NOT  AllPortsSameDT=off  OutDataTypeStr=boolean
  NOT1 : Logic  Operator=NOT  AllPortsSameDT=off  OutDataTypeStr=boolean
  NOT2 : Logic  Operator=NOT  AllPortsSameDT=off  OutDataTypeStr=boolean
  Product : Product
  Product1 : Product
  Product2 : Product
  Scope : Scope  NumInputPorts=2
  Scope1 : Scope  NumInputPorts=3
  Scope2 : Scope  NumInputPorts=3
  Scope3 : Scope  NumInputPorts=3
  Scope4 : Scope  NumInputPorts=4
  Traingle1 : simulink/Sources/Repeating Sequence  rep_seq_t=[0 1/20000]  rep_seq_y=[-100 100]
  alpha-beta to ABC : Subsystem
  g1 : Outport
  g4 : Outport  Port=2
  g3 : Outport  Port=3
  g6 : Outport  Port=4
  g5 : Outport  Port=5
  g2 : Outport  Port=6
  gate : Outport  Port=7
  wires:
  Compare To Zero2/1 -> Mux1/5, g5/1, NOT2/1
  Compare To Zero/1 -> Mux1/1, g1/1, Scope/2, NOT/1
  Mux/1 -> Scope/1
  alpha-beta to ABC/1(Va) -> Product/2, Scope1/1, Mux/1, Add/1
  Add/1 -> Compare To Zero/1
  Add2/1 -> Compare To Zero2/1
  Compare To Zero1/1 -> Mux1/3, g3/1, NOT1/1
  Traingle1/1 -> Mux/2, Add/2, Add1/2, Add2/2
  Add1/1 -> Compare To Zero1/1
  alpha_beta/1 -> alpha-beta to ABC/1(alpha_beta)
  NOT1/1 -> Mux1/4, g6/1
  alpha-beta to ABC/2(Vb) -> Add1/1, Product1/2, Scope1/2
  alpha-beta to ABC/3(Vc) -> Product2/2, Scope1/3, Add2/1
  NOT/1 -> Mux1/2, g4/1
  NOT2/1 -> Mux1/6, g2/1
  Mux1/1 -> gate/1
  Demux/1 -> Scope4/1, Scope2/1, Product/1
  [hall] -> Demux/1
  Demux/2 -> Scope4/3, Product1/1, Scope2/3
  Demux/3 -> Scope2/2, Product2/1
  Product/1 -> Scope3/1
  Product1/1 -> Scope3/2
  Product2/1 -> Scope3/3
  [Ea] -> Scope4/2
  [Eb] -> Scope4/4

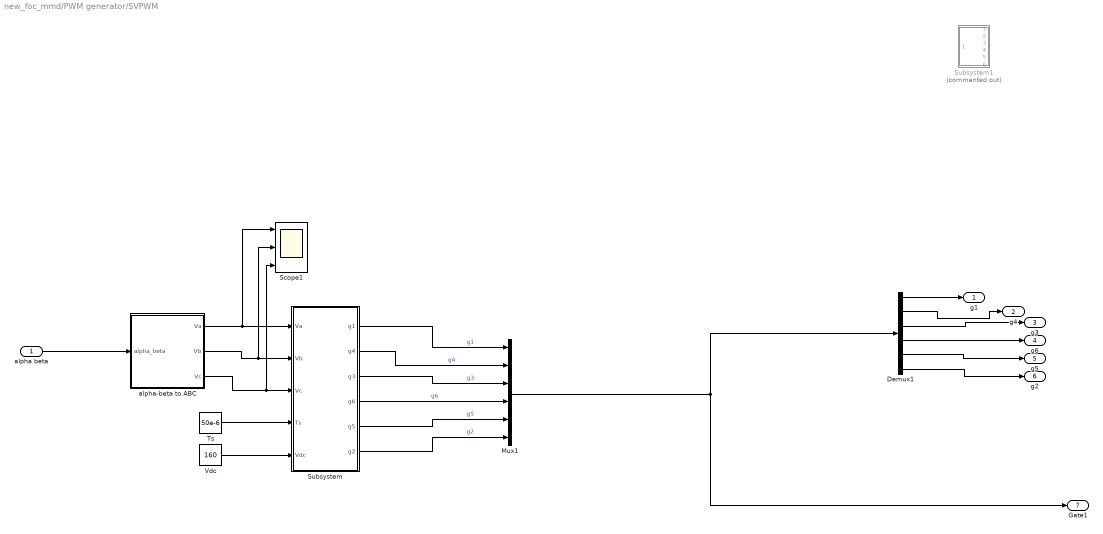
== system new_foc_mmd/PWM generator/SVPWM ==
  alpha beta : Inport
  Demux1 : Demux  Outputs=6
  Mux1 : Mux  Inputs=6
  Scope1 : Scope  NumInputPorts=3
  Subsystem : Subsystem
  Subsystem1 : Subsystem  Commented=on
  Ts : Constant  Value=50e-6
  Vdc : Constant  Value=160
  alpha-beta to ABC : Subsystem
  g1 : Outport
  g4 : Outport  Port=2
  g3 : Outport  Port=3
  g6 : Outport  Port=4
  g5 : Outport  Port=5
  g2 : Outport  Port=6
  Gate1 : Outport  Port=7
  wires:
  Vdc/1 -> Subsystem/5(Vdc)
  Ts/1 -> Subsystem/4(Ts)
  alpha beta/1 -> alpha-beta to ABC/1(alpha_beta)
  alpha-beta to ABC/1(Va) -> Scope1/1, Subsystem/1(Va)
  alpha-beta to ABC/2(Vb) -> Scope1/2, Subsystem/2(Vb)
  alpha-beta to ABC/3(Vc) -> Scope1/3, Subsystem/3(Vc)
  Demux1/5 -> g5/1
  Demux1/4 -> g6/1
  Demux1/2 -> g4/1
  Demux1/3 -> g3/1
  Subsystem/4(g6) -> Mux1/4  "g6"
  Subsystem/2(g4) -> Mux1/2  "g4"
  Subsystem/5(g5) -> Mux1/5  "g5"
  Demux1/1 -> g1/1
  Subsystem/6(g2) -> Mux1/6  "g2"
  Mux1/1 -> Demux1/1, Gate1/1
  Subsystem/3(g3) -> Mux1/3  "g3"
  Demux1/6 -> g2/1
  Subsystem/1(g1) -> Mux1/1  "g1"

== system new_foc_mmd/BLDC Model3/Generation of Signal For Hall Effect Sensors/theta_elec to theta_degree ==
  theta_elec : Inport
  Trigonometric Function : Trigonometry
  Trigonometric Function1 : Trigonometry  Operator=cos
  Trigonometric Function2 : Trigonometry  Operator=atan2
  rad to deg : Gain  Gain=180/pi  SaturateOnIntegerOverflow=on  OutDataTypeStr=Inherit: Same as input  ParamDataTypeStr=Inherit: Same as input
  theta_degree : Outport
  wires:
  Trigonometric Function2/1 -> rad to deg/1
  Trigonometric Function/1 -> Trigonometric Function2/1
  Trigonometric Function1/1 -> Trigonometric Function2/2
  theta_elec/1 -> Trigonometric Function1/1, Trigonometric Function/1
  rad to deg/1 -> theta_degree/1

== system new_foc_mmd/PWM generator/PWM/Gate Pulse ==
  gates : Inport
  Compare To Zero : simulink/Logic and Bit Operations/Compare To Zero  relop=>  OutDataTypeStr=boolean
  Compare To Zero1 : simulink/Logic and Bit Operations/Compare To Zero  relop=>  OutDataTypeStr=boolean
  Compare To Zero2 : simulink/Logic and Bit Operations/Compare To Zero  relop=>  OutDataTypeStr=boolean
  Compare To Zero3 : simulink/Logic and Bit Operations/Compare To Zero  relop=<  OutDataTypeStr=boolean
  Compare To Zero4 : simulink/Logic and Bit Operations/Compare To Zero  relop=<  OutDataTypeStr=boolean
  Compare To Zero5 : simulink/Logic and Bit Operations/Compare To Zero  relop=<  OutDataTypeStr=boolean
  Demux : Demux  Outputs=3
  Mux : Mux  Inputs=6
  Out1 : Outport
  wires:
  Compare To Zero1/1 -> Mux/3
  Demux/2 -> Compare To Zero4/1, Compare To Zero1/1
  Compare To Zero3/1 -> Mux/2
  Demux/3 -> Compare To Zero5/1, Compare To Zero2/1
  Compare To Zero2/1 -> Mux/5
  Demux/1 -> Compare To Zero3/1, Compare To Zero/1
  Compare To Zero4/1 -> Mux/4
  Compare To Zero5/1 -> Mux/6
  Compare To Zero/1 -> Mux/1
  gates/1 -> Demux/1
  Mux/1 -> Out1/1

== system new_foc_mmd/PWM generator/PWM/alpha-beta to ABC ==
  alpha_beta : Inport
  Demux : Demux  Outputs=2
  Gain5 : Gain  Gain=2/3
  Gain6 : Gain  Gain=1/sqrt(3)
  Gain7 : Gain  Gain=-1/3
  Gain8 : Gain  Gain=-1/3
  Gain9 : Gain  Gain=-1/sqrt(3)
  Sum1 : Sum  Inputs=|++
  Sum2 : Sum  Inputs=|++
  Va : Outport
  Vb : Outport  Port=2
  Vc : Outport  Port=3
  wires:
  Demux/1 -> Gain5/1, Gain8/1, Gain7/1
  Gain5/1 -> Va/1
  Demux/2 -> Gain9/1, Gain6/1
  Gain6/1 -> Sum1/1
  Gain7/1 -> Sum1/2
  Sum1/1 -> Vb/1
  Gain8/1 -> Sum2/1
  Gain9/1 -> Sum2/2
  Sum2/1 -> Vc/1
  alpha_beta/1 -> Demux/1

== system new_foc_mmd/PWM generator/SPWM/alpha-beta to ABC ==
  alpha_beta : Inport
  Demux : Demux  Outputs=2
  Gain5 : Gain  Gain=2/3
  Gain6 : Gain  Gain=1/sqrt(3)
  Gain7 : Gain  Gain=-1/3
  Gain8 : Gain  Gain=-1/3
  Gain9 : Gain  Gain=-1/sqrt(3)
  Sum1 : Sum  Inputs=|++
  Sum2 : Sum  Inputs=|++
  Va : Outport
  Vb : Outport  Port=2
  Vc : Outport  Port=3
  wires:
  Demux/1 -> Gain5/1, Gain8/1, Gain7/1
  Gain5/1 -> Va/1
  Demux/2 -> Gain9/1, Gain6/1
  Gain6/1 -> Sum1/1
  Gain7/1 -> Sum1/2
  Sum1/1 -> Vb/1
  Gain8/1 -> Sum2/1
  Gain9/1 -> Sum2/2
  Sum2/1 -> Vc/1
  alpha_beta/1 -> Demux/1

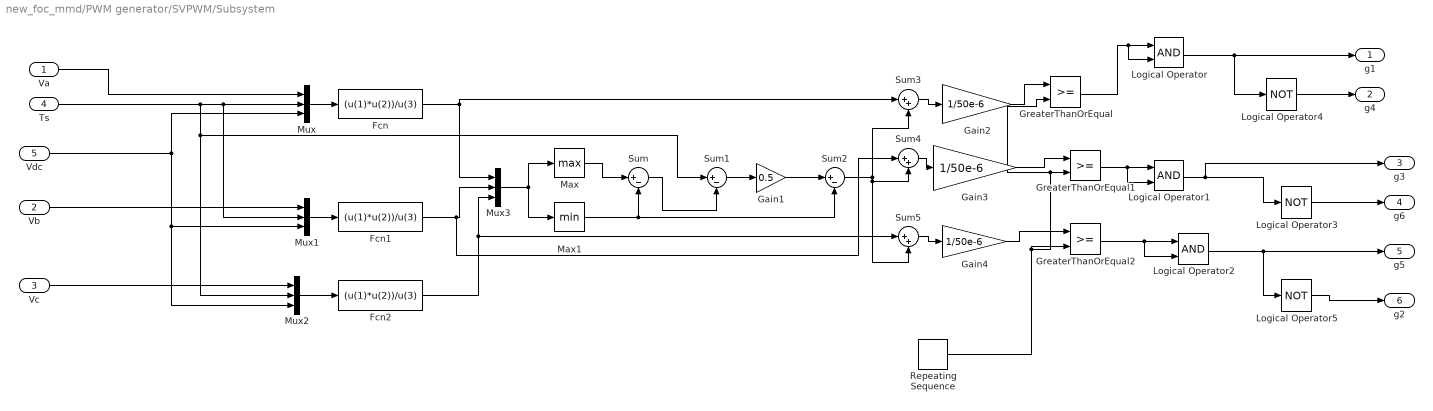
== system new_foc_mmd/PWM generator/SVPWM/Subsystem ==
  Va : Inport
  Vb : Inport  Port=2
  Vc : Inport  Port=3
  Ts : Inport  Port=4
  Vdc : Inport  Port=5
  Fcn : Fcn  Expr=(u(1)*u(2))/u(3)
  Fcn1 : Fcn  Expr=(u(1)*u(2))/u(3)
  Fcn2 : Fcn  Expr=(u(1)*u(2))/u(3)
  Gain1 : Gain  Gain=0.5
  Gain2 : Gain  Gain=1/50e-6
  Gain3 : Gain  Gain=1/50e-6
  Gain4 : Gain  Gain=1/50e-6
  GreaterThanOrEqual : RelationalOperator  OutDataTypeStr=boolean  RndMeth=Simplest  InputSameDT=off
  GreaterThanOrEqual1 : RelationalOperator  OutDataTypeStr=boolean  RndMeth=Simplest  InputSameDT=off
  GreaterThanOrEqual2 : RelationalOperator  OutDataTypeStr=boolean  RndMeth=Simplest  InputSameDT=off
  Logical Operator : Logic  AllPortsSameDT=off  OutDataTypeStr=boolean
  Logical Operator1 : Logic  AllPortsSameDT=off  OutDataTypeStr=boolean
  Logical Operator2 : Logic  AllPortsSameDT=off  OutDataTypeStr=boolean
  Logical Operator3 : Logic  Operator=NOT  AllPortsSameDT=off  OutDataTypeStr=boolean
  Logical Operator4 : Logic  Operator=NOT  AllPortsSameDT=off  OutDataTypeStr=boolean
  Logical Operator5 : Logic  Operator=NOT  AllPortsSameDT=off  OutDataTypeStr=boolean
  Max : MinMax  Function=max
  Max1 : MinMax
  Mux{,1..3} (4 alike) : Mux  Inputs=3
  Repeating Sequence : simulink/Sources/Repeating Sequence  rep_seq_t=[0 0.25 0.5 0.75 1]/1250  rep_seq_y=[1 0 -1 0 1]
  Sum : Sum  Inputs=|+-
  Sum1 : Sum  Inputs=|+-
  Sum2 : Sum  Inputs=|+-
  Sum3 : Sum  Inputs=|++
  Sum4 : Sum  Inputs=|++
  Sum5 : Sum  Inputs=|++
  g1 : Outport
  g4 : Outport  Port=2
  g3 : Outport  Port=3
  g6 : Outport  Port=4
  g5 : Outport  Port=5
  g2 : Outport  Port=6
  wires:
  Ts/1 -> Sum1/1, Mux2/2, Mux1/2, Mux/2
  GreaterThanOrEqual1/1 -> Logical Operator1/2, Logical Operator1/1
  Sum2/1 -> Sum5/2, Sum4/2, Sum3/2
  Logical Operator1/1 -> Logical Operator3/1, g3/1
  Vdc/1 -> Mux/3, Mux1/3, Mux2/3
  Logical Operator4/1 -> g4/1
  Logical Operator2/1 -> g5/1, Logical Operator5/1
  Sum5/1 -> Gain4/1
  Repeating Sequence/1 -> GreaterThanOrEqual/2, GreaterThanOrEqual1/2, GreaterThanOrEqual2/2
  Logical Operator/1 -> g1/1, Logical Operator4/1
  Fcn/1 -> Sum3/1, Mux3/1
  Sum3/1 -> Gain2/1
  Gain4/1 -> GreaterThanOrEqual2/1
  Gain2/1 -> GreaterThanOrEqual/1
  Gain1/1 -> Sum2/1
  Mux3/1 -> Max/1, Max1/1
  Sum4/1 -> Gain3/1
  GreaterThanOrEqual/1 -> Logical Operator/2, Logical Operator/1
  Vb/1 -> Mux1/1
  Fcn2/1 -> Sum5/1, Mux3/3
  Fcn1/1 -> Sum4/1, Mux3/2
  Vc/1 -> Mux2/1
  GreaterThanOrEqual2/1 -> Logical Operator2/2, Logical Operator2/1
  Max/1 -> Sum/1
  Mux2/1 -> Fcn2/1
  Mux1/1 -> Fcn1/1
  Sum1/1 -> Gain1/1
  Mux/1 -> Fcn/1
  Va/1 -> Mux/1
  Max1/1 -> Sum2/2, Sum/2
  Sum/1 -> Sum1/2
  Gain3/1 -> GreaterThanOrEqual1/1
  Logical Operator3/1 -> g6/1
  Logical Operator5/1 -> g2/1

== system new_foc_mmd/PWM generator/SVPWM/Subsystem1 ==
  alpha beta : Inport
  Demux : Demux  Commented=on  Outputs=6
  Mux4 : Mux  Commented=on  Inputs=6
  Space Vector PWM : Subsystem  Commented=on
  Out1 : Outport
  Out2 : Outport  Port=2
  Out3 : Outport  Port=3
  Out4 : Outport  Port=4
  Out5 : Outport  Port=5
  Out6 : Outport  Port=6
  wires:
  Space Vector PWM/6(Vg2) -> Mux4/6  "g2"
  Mux4/1 -> Demux/1
  Demux/1 -> Out1/1
  Space Vector PWM/1(Vg1) -> Mux4/1  "g1"
  Space Vector PWM/3(Vg3) -> Mux4/3  "g3"
  Space Vector PWM/4(Vg6) -> Mux4/4  "g6"
  Space Vector PWM/2(Vg4) -> Mux4/2  "g4"
  alpha beta/1 -> Space Vector PWM/1(alpha beta)
  Demux/3 -> Out3/1
  Space Vector PWM/5(Vg5) -> Mux4/5  "g5"
  Demux/2 -> Out2/1
  Demux/5 -> Out5/1
  Demux/4 -> Out4/1
  Demux/6 -> Out6/1

== system new_foc_mmd/PWM generator/SVPWM/alpha-beta to ABC ==
  alpha_beta : Inport
  Demux : Demux  Outputs=2
  Gain5 : Gain  Gain=2/3
  Gain6 : Gain  Gain=1/sqrt(3)
  Gain7 : Gain  Gain=-1/3
  Gain8 : Gain  Gain=-1/3
  Gain9 : Gain  Gain=-1/sqrt(3)
  Scope : Scope  NumInputPorts=3
  Sum1 : Sum  Inputs=|++
  Sum2 : Sum  Inputs=|++
  Va : Outport
  Vb : Outport  Port=2
  Vc : Outport  Port=3
  wires:
  Demux/1 -> Gain5/1, Gain8/1, Gain7/1
  Gain5/1 -> Scope/1, Va/1
  Demux/2 -> Gain9/1, Gain6/1
  Gain6/1 -> Sum1/1
  Gain7/1 -> Sum1/2
  Sum1/1 -> Scope/2, Vb/1
  Gain8/1 -> Sum2/1
  Gain9/1 -> Sum2/2
  Sum2/1 -> Scope/3, Vc/1
  alpha_beta/1 -> Demux/1

== system new_foc_mmd/PWM generator/SVPWM/Subsystem1/Space Vector PWM ==
  alpha beta : Inport
  Demux : Demux  Outputs=2
  Fcn : Fcn  Expr=floor(u/60)+1
  Gate signals : Subsystem
  Modulation index : Subsystem
  T0_T1_T2 : Subsystem
  Ts : Constant  Value=Ts
  Vref and angle calclator : Subsystem
  Vg1 : Outport  VectorParamsAs1DForOutWhenUnconnected=off
  Vg4 : Outport  Port=2  VectorParamsAs1DForOutWhenUnconnected=off
  Vg3 : Outport  Port=3  VectorParamsAs1DForOutWhenUnconnected=off
  Vg6 : Outport  Port=4  VectorParamsAs1DForOutWhenUnconnected=off
  Vg5 : Outport  Port=5  VectorParamsAs1DForOutWhenUnconnected=off
  Vg2 : Outport  Port=6  VectorParamsAs1DForOutWhenUnconnected=off
  wires:
  Fcn/1 -> T0_T1_T2/2(n), Gate signals/5(n)
  T0_T1_T2/3(T2) -> Gate signals/3(T2)
  Demux/2 -> Vref and angle calclator/2(Vbeta)
  Gate signals/5(Vg5) -> Vg5/1
  Gate signals/4(Vg6) -> Vg6/1
  Gate signals/2(Vg4) -> Vg4/1
  Gate signals/3(Vg3) -> Vg3/1
  Gate signals/1(Vg1) -> Vg1/1
  Ts/1 -> Gate signals/4(Ts), T0_T1_T2/4(Ts)
  Gate signals/6(Vg2) -> Vg2/1
  T0_T1_T2/1(T0) -> Gate signals/1(T0)
  T0_T1_T2/2(T1) -> Gate signals/2(T1)
  Vref and angle calclator/2(Vref) -> Modulation index/1(Vref)
  Modulation index/1(a) -> T0_T1_T2/3(a)
  Vref and angle calclator/1(alpha) -> Fcn/1, T0_T1_T2/1(alpha)
  alpha beta/1 -> Demux/1
  Demux/1 -> Vref and angle calclator/1(Valpha)
